simulink model "untitled"  (R2015a)
settings: Solver=ode45  StartTime=0.0  StopTime=2  RelTol=1e-3
libraries: commutil2 x2, dspquant2 x2, commchan3 x1, dspmlti4 x1
settings Model: Creator=student  LastModifiedBy=student

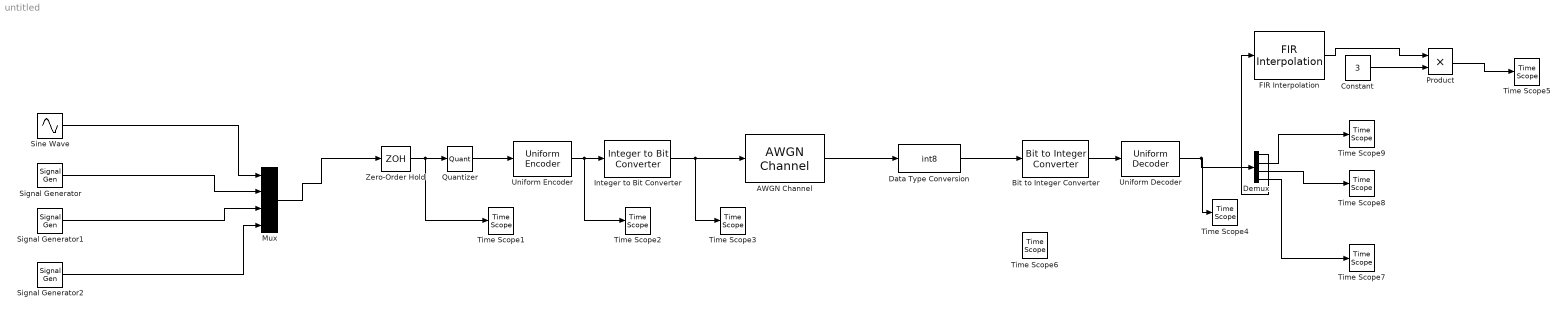
== system untitled ==
  AWGN Channel : commchan3/AWGN Channel  InputProcessing=Columns as channels (frame based)  seed=67  noiseMode="Signal to noise ratio  (Eb/No)"  EbNodB=300  EsNodB=10  SNRdB=10  bitsPerSym=16  Ps=0.01  Tsym=1/(1500*2*pi)  variance=1
  Bit to Integer Converter : commutil2/Bit to Integer Converter  nbits=8  bitOrder=MSB first  signedOutputValues=Signed  outDtype=int8  outDtypeSigned=Inherit via internal rule
  Constant : Constant  Value=3
  Data Type Conversion : DataTypeConversion  OutMin=[0]  OutMax=[1]  OutDataTypeStr=int8  RndMeth=Zero
  Demux : Demux
  FIR Interpolation : dspmlti4/FIR Interpolation  h=fir1(13,1/4)  L=3  framing=Enforce single-rate processing  outputBufInitCond=0  InputProcessing=Columns as channels (frame based)  firstCoeffDataTypeStr=Inherit: Same word length as input  firstCoeffLastDataTypeStr=Inherit: Same word length as input  firstCoeffMin=[]  firstCoeffMax=[]  outputDataTypeStr=Inherit: Same as accumulator  outputLastDataTypeStr=Inherit: Same as accumulator  outputMin=[]  outputMax=[]  roundingMode=Floor  overflowMode=on  FilterSource=Specify via dialog  FilterObject=Hm_firinterp
  Integer to Bit Converter : commutil2/Integer to Bit Converter  nbits=8  signedInputValues=Signed  bitOrder=MSB first  outDtype=double
  Mux : Mux
  Product : Product
  Quantizer : Quantizer
  Signal Generator : SignalGenerator  WaveForm=square  Amplitude=3  Frequency=500
  Signal Generator1 : SignalGenerator  WaveForm=sawtooth  Amplitude=3  Frequency=500
  Signal Generator2 : SignalGenerator  WaveForm=random  Amplitude=3  Frequency=500
  Sine Wave : Sin  Amplitude=3  Frequency=1500*2*pi  SampleTime=1/80000
  Time Scope{1..9} (9 alike) : TimeScope  DefaultConfigurationName=spbscopes.TimeScopeBlockCfg
  Uniform Decoder : dspquant2/Uniform Decoder  peak=3  bits=8  overflowMode=Saturate  otype=Double
  Uniform Encoder : dspquant2/Uniform Encoder  peak=3  bits=8  otype=Signed integer
  Zero-Order Hold : ZeroOrderHold  SampleTime=1/8000
  wires:
  Quantizer/1 -> Uniform Encoder/1
  Zero-Order Hold/1 -> Time Scope1/1, Quantizer/1
  Uniform Encoder/1 -> Time Scope2/1, Integer to Bit Converter/1
  Bit to Integer Converter/1 -> Uniform Decoder/1
  Uniform Decoder/1 -> Demux/1, Time Scope4/1
  FIR Interpolation/1 -> Product/1
  Constant/1 -> Product/2
  Integer to Bit Converter/1 -> AWGN Channel/1, Time Scope3/1
  AWGN Channel/1 -> Data Type Conversion/1
  Data Type Conversion/1 -> Bit to Integer Converter/1
  Sine Wave/1 -> Mux/1
  Signal Generator/1 -> Mux/2
  Signal Generator1/1 -> Mux/3
  Signal Generator2/1 -> Mux/4
  Demux/2 -> Time Scope9/1
  Mux/1 -> Zero-Order Hold/1
  Demux/3 -> Time Scope8/1
  Demux/4 -> Time Scope7/1
  Product/1 -> Time Scope5/1
  Demux/1 -> FIR Interpolation/1
